simulink model "speed2"  (R2017b)
settings: Solver=ode5  StartTime=0.0  StopTime=20  FixedStep=0.0001  RelTol=1e-3  EnableMultiTasking=on
libraries: slrtlib x5, xpcnilib x4, dspswit3 x3, dspsigops x3, simulink x1, simulink_extras x1
settings Model: SimulationMode=external  Creator=Lab322  LastModifiedBy=nimaaghli
settings DataIOCC: MaxDataPoints=10000  SaveFormat=Array
settings OptimizationCC: BlockReduction=off  OptimizeBlockIOStorage=off  BufferReuse=off  GlobalBufferReuse=off  ExpressionFolding=off  LocalBlockOutputs=off  LifeSpan=inf
settings DebuggingCC: SolverPrmCheckMsg=warning  SFUnexpectedBacktrackingDiag=warning  SFNoUnconditionalDefaultTransitionDiag=warning  SFExecutionAtInitializationDiag=none
settings HardwareCC: ProdBitPerPointer=32  ProdBitPerSizeT=32  ProdBitPerPtrDiffT=32  ProdLargestAtomicFloat=None  ProdWordSize=32  ProdHWDeviceType=Generic->32-bit x86 compatible
settings ModelReferenceCC: PropagateSignalLabelsOutOfModel=off
settings RTWCC: SystemTargetFile=slrt.tlc  TemplateMakefile=slrt_default_tmf  Description=Simulink Real-Time  RTWCompilerOptimization=on
settings CodeAppCC: StateflowObjectComments=on
settings TargetCC: CodeReplacementLibrary=XPC_BLAS  ParMdlRefBuildCompliant=on  ConcurrentExecutionCompliant=on  MatFileLogging=on  MATLABClassNameForMDSCustomization=xpcAperiodicCustomization
settings ConfigComp: CovMetricSettings=dw  CovHtmlReporting=on  CovSaveCumulativeToWorkspaceVar=on  CovSaveSingleToWorkspaceVar=on  CovExternalEMLEnable=off  CovSFcnEnable=off
settings SimscapeCC: SimscapeNormalizeSystem=off
settings ConfigurationSet: Description=SimMechanics 2G

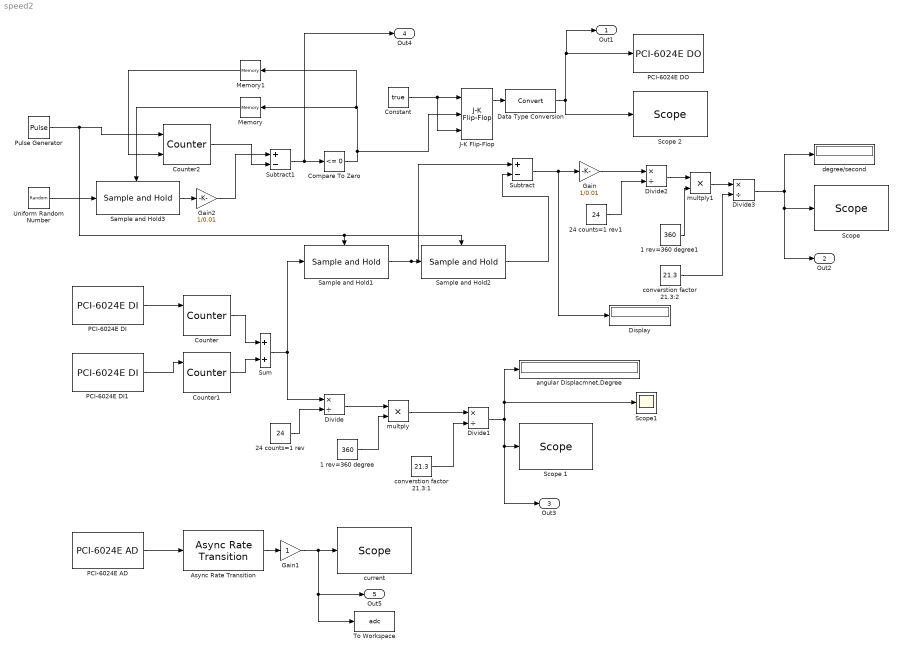
== system speed2 ==
  1 rev=360 degree : Constant  Value=360
  1 rev=360 degree1 : Constant  Value=360
  24 counts=1 rev : Constant  Value=24
  24 counts=1 rev1 : Constant  Value=24
  "Async Rate Transition " : slrtlib/Asynchronous Event/Async Rate Transition   sample_time=0.001
      settings: SourceProductName=Simulink Real-Time  SourceProductBaseCode=XP
  Compare To Zero : simulink/Logic and Bit Operations/Compare To Zero  relop=<=  OutDataTypeStr=boolean
  Constant : Constant  Value=true
  Counter : dspswit3/Counter  Direction=Up  CountEvent=Rising edge  CounterSize=User defined  MaxCount=10000000  InitialCount=0  Output=Count  HitValue=32  ResetInput=on  SamplesPerFrame=1  Ts=1  CntDtype=double  HitDtype=Logical
  Counter1 : dspswit3/Counter  Direction=Up  CountEvent=Rising edge  CounterSize=User defined  MaxCount=10000000  InitialCount=0  Output=Count  HitValue=32  ResetInput=on  SamplesPerFrame=1  Ts=1  CntDtype=double  HitDtype=Logical
  Counter2 : dspswit3/Counter  Direction=Up  CountEvent=Rising edge  CounterSize=User defined  MaxCount=100000000  InitialCount=0  Output=Count  HitValue=32  ResetInput=on  SamplesPerFrame=1  Ts=1  CntDtype=double  HitDtype=Logical
  Data Type Conversion : DataTypeConversion
  Display : Display
  Divide{,1..3} (4 alike) : Product  Inputs=*/
  Gain : Gain  Gain=1/0.01
  Gain1 : Gain
  Gain2 : Gain  Gain=1/0.01
  J-K Flip-Flop : simulink_extras/Flip Flops/J-K Flip-Flop  initial_condition=0
      settings: SourceProductName=Simulink
  Memory : Memory
  Memory1 : Memory
  PCI-6024E AD : xpcnilib/A//D/E Series/PCI-6024E AD  channel=[1]  range=[-10]  coupling=[0]  sampletime=0.0001  slot=-1
      settings: SourceProductName=Simulink Real-Time  SourceProductBaseCode=XP
  PCI-6024E DI : xpcnilib/Digital Input/E Series/PCI-6024E DI  channel=[7]  sampletime=0.0001  slot=-1
      settings: SourceProductName=Simulink Real-Time  SourceProductBaseCode=XP
  PCI-6024E DI1 : xpcnilib/Digital Input/E Series/PCI-6024E DI  channel=[8]  sampletime=0.0001  slot=-1
      settings: SourceProductName=Simulink Real-Time  SourceProductBaseCode=XP
  PCI-6024E DO : xpcnilib/Digital Output/E Series/PCI-6024E DO  channel=[3]  reset=[1]  initValue=[0]  sampletime=0.0001  slot=-1
      settings: SourceProductName=Simulink Real-Time  SourceProductBaseCode=XP
  Pulse Generator : DiscretePulseGenerator  PulseType=Time based  Period=0.01  PulseWidth=50
  Sample and Hold1 : dspsigops/Sample and Hold  trig=Rising edge  initCond=0  latchinput=on
  Sample and Hold2 : dspsigops/Sample and Hold  trig=Rising edge  initCond=0  latchinput=on
  Sample and Hold3 : dspsigops/Sample and Hold  trig=Rising edge  initCond=2  latchinput=off
  "Scope " : slrtlib/Displays and Logging/Scope   scopeno=1  scopetype=Target  autostart=on  viewmode=Graphical redraw  formatstr='%15.6f'  grid=on  ylimits=[0,0]  nosamples=250  noprepostsamples=0  interleave=1  triggermode=FreeRun  triggersignal=1  trigsignalfromport=off  triggerlevel=0.0  triggerslope=Either  triggerscope=1  triggersample=0  filename=data.dat  mode=Lazy  writesize=512  autorestart=off  dynamicfilemode=off  maxwritefilesize=512*1024^2
  Scope 1 : slrtlib/Displays and Logging/Scope   scopeno=3  scopetype=Target  autostart=on  viewmode=Graphical redraw  formatstr='%15.6f'  grid=on  ylimits=[0,0]  nosamples=600  noprepostsamples=0  interleave=1  triggermode=FreeRun  triggersignal=1  trigsignalfromport=off  triggerlevel=0.0  triggerslope=Either  triggerscope=1  triggersample=0  filename=data.dat  mode=Lazy  writesize=512  autorestart=off  dynamicfilemode=off  maxwritefilesize=512*1024^2
  Scope 2 : slrtlib/Displays and Logging/Scope   scopeno=4  scopetype=Target  autostart=on  viewmode=Graphical redraw  formatstr='%15.6f'  grid=on  ylimits=[0,0]  nosamples=600  noprepostsamples=0  interleave=1  triggermode=FreeRun  triggersignal=1  trigsignalfromport=off  triggerlevel=0.0  triggerslope=Either  triggerscope=1  triggersample=0  filename=data.dat  mode=Lazy  writesize=512  autorestart=off  dynamicfilemode=off  maxwritefilesize=512*1024^2
  Scope1 : Scope
  Subtract : Sum  Inputs=+-
  Subtract1 : Sum  Inputs=+-
  Sum : Sum
  To Workspace : ToWorkspace  VariableName=adc  SampleTime=-1
  Uniform Random Number : UniformRandomNumber  Minimum=0  SampleTime=0.0001
  angular Displacmnet,Degree : Display
  converstion factor 21.3:1 : Constant  Value=21.3
  converstion factor 21.3:2 : Constant  Value=21.3
  current : slrtlib/Displays and Logging/Scope   scopeno=2  scopetype=Target  autostart=on  viewmode=Graphical redraw  formatstr='%15.6f'  grid=on  ylimits=[0,0]  nosamples=60000  noprepostsamples=0  interleave=1  triggermode=FreeRun  triggersignal=1  trigsignalfromport=off  triggerlevel=0.0  triggerslope=Either  triggerscope=1  triggersample=0  filename=data.dat  mode=Lazy  writesize=512  autorestart=off  dynamicfilemode=off  maxwritefilesize=512*1024^2
  degree/second : Display
  multply : Product  Inputs=**
  multply1 : Product  Inputs=**
  Out1 : Outport
  Out2 : Outport  Port=2
  Out3 : Outport  Port=3
  Out4 : Outport  Port=4
  Out5 : Outport  Port=5
  wires:
  PCI-6024E DI/1 -> Counter/1
  Sample and Hold1/1 -> Subtract/1, Sample and Hold2/1
  Sample and Hold2/1 -> Subtract/2
  PCI-6024E DI1/1 -> Counter1/1
  Sum/1 -> Divide/1, Sample and Hold1/1
  Counter/1 -> Sum/1
  Counter1/1 -> Sum/2
  Subtract/1 -> Display/1, Gain/1
  24 counts=1 rev/1 -> Divide/2
  converstion factor 21.3:1/1 -> Divide1/2
  multply/1 -> Divide1/1
  Divide/1 -> multply/1
  1 rev=360 degree/1 -> multply/2
  Divide1/1 -> angular Displacmnet,Degree/1, Scope1/1, Out3/1, Scope 1/1
  24 counts=1 rev1/1 -> Divide2/2
  converstion factor 21.3:2/1 -> Divide3/2
  multply1/1 -> Divide3/1
  Divide2/1 -> multply1/1
  1 rev=360 degree1/1 -> multply1/2
  Gain/1 -> Divide2/1
  Divide3/1 -> degree/second/1, Out2/1, "Scope "/1
  PCI-6024E AD/1 -> "Async Rate Transition "/1
  "Async Rate Transition "/1 -> Gain1/1
  Gain1/1 -> Out5/1, To Workspace/1, current/1
  Pulse Generator/1 -> Sample and Hold2/Trigger, Sample and Hold1/Trigger, Counter2/1
  Uniform Random Number/1 -> Sample and Hold3/1
  Subtract1/1 -> Out4/1, Compare To Zero/1
  Compare To Zero/1 -> J-K Flip-Flop/2, Memory1/1, Memory/1
  Sample and Hold3/1 -> Gain2/1
  Gain2/1 -> Subtract1/1
  Memory/1 -> Sample and Hold3/Trigger
  Counter2/1 -> Subtract1/2
  Memory1/1 -> Counter2/2
  J-K Flip-Flop/1 -> Data Type Conversion/1
  Constant/1 -> J-K Flip-Flop/3, J-K Flip-Flop/1
  Data Type Conversion/1 -> PCI-6024E DO/1, Out1/1, Scope 2/1
